simulink model "mc2_current"  (R2023b)
settings: Solver=ode45  StartTime=0.0  StopTime=0.05  MaxStep=1e-5  RelTol=1e-3
libraries: simulink x1, spsDCVoltageSourceLib x1, spsUniversalBridgeLib x1, spsVoltageMeasurementLib x1, sps_lib x1
settings Model: Creator=86189  LastModifiedBy=86189

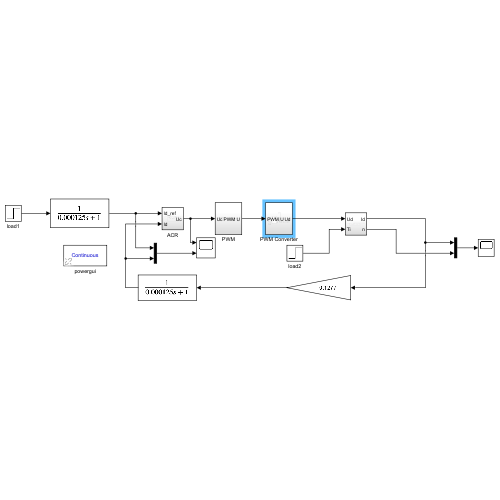
[thumbnail: Simulink's stored preview of the top-level diagram]
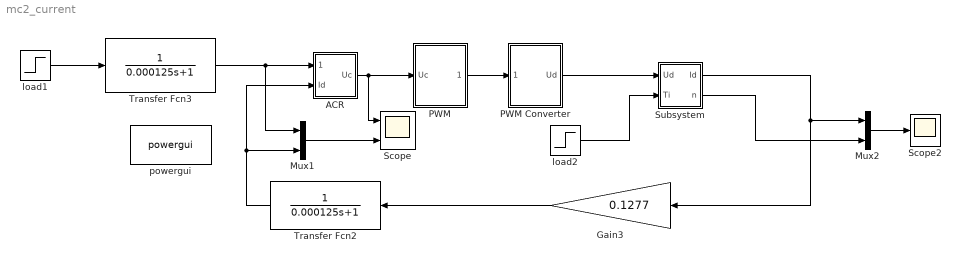
== system mc2_current ==
  ACR : Subsystem
  Gain3 : Gain  Gain=0.1277
  Mux1 : Mux  Inputs=2
  Mux2 : Mux  Inputs=2
  PWM : Subsystem
  PWM Converter : Subsystem
  Scope : Scope  NumInputPorts=2
  Scope2 : Scope
  Subsystem : Subsystem
  Transfer Fcn2 : TransferFcn  Denominator=[0.000125 1]
  Transfer Fcn3 : TransferFcn  Denominator=[0.000125 1]
  load1 : Step  Time=0  After=10  SampleTime=0
  load2 : Step  Time=0  After=10  SampleTime=0
  powergui : sps_lib/powergui  Priority=1  SimulationMode=Continuous  SampleTime=50e-6  frequency=60  Iterations=50  frequencyindice=0  Pbase=100e6  ErrMax=1e-4  UnitsV=kV  UnitsW=MW  buscounter=0  FunctionMessages=off  echomessages=off  EnableUseOfTLC=off  CurrentSourceSwitches=off  DisableSnubberDevices=off  DisableRonSwitches=off  DisableVfSwitches=off  DisplayEquations=off  AutomaticDiscreteSolvers=off  SolverType=Tustin/Backward Euler (TBE)  Interpol=off  ExternalGateDelay=off  methode=off  Ts=100  x0status=blocks  SPID=on  SwTol=0  HookPort=off  NonlinearTolerance=1e-4  nMaxIteration=100  ContinueOnMaxIteration=off  RestoreLinks=warning  ResistiveCurrentMeasurement=off  Frange=[0:2:500]  Ylog=off  Xlog=on  ShowGrid=off  save=off  variable=ZData  structure=0  ZoomFFT=off  StartTime=0.0  cycles=1  DisplayStyle=1  fundamental=60  FreqAxis=off  MaxFrequency=1000  frequencyindicesteady=1  RmsSteady=1  display=off
  wires:
  load1/1 -> Transfer Fcn3/1
  Gain3/1 -> Transfer Fcn2/1
  PWM Converter/1(Ud) -> Subsystem/1(Ud)
  Subsystem/1(Id) -> Mux2/1, Gain3/1
  load2/1 -> Subsystem/2(Ti)
  PWM/1(PWM U) -> PWM Converter/1(PWM U)
  Transfer Fcn3/1 -> Mux1/1, ACR/1(Id_ref)
  Transfer Fcn2/1 -> Mux1/2, ACR/2(Id)
  ACR/1(Uc) -> Scope/1, PWM/1(Uc)
  Mux1/1 -> Scope/2
  Subsystem/2(n) -> Mux2/2
  Mux2/1 -> Scope2/1

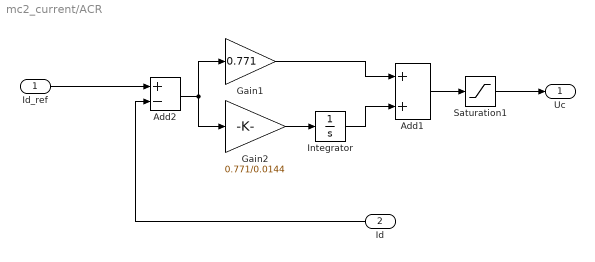
== system mc2_current/ACR ==
  Id_ref : Inport
  Id : Inport  Port=2
  Add1 : Sum
  Add2 : Sum  Inputs=+-
  Gain1 : Gain  Gain=0.771
  Gain2 : Gain  Gain=0.771/0.0144
  Integrator : Integrator  LimitOutput=on  UpperSaturationLimit=5  LowerSaturationLimit=-5
  Saturation1 : Saturate  UpperLimit=5  LowerLimit=-5
  Uc : Outport
  wires:
  Gain2/1 -> Integrator/1
  Add1/1 -> Saturation1/1
  Integrator/1 -> Add1/2
  Add2/1 -> Gain2/1, Gain1/1
  Gain1/1 -> Add1/1
  Id/1 -> Add2/2
  Id_ref/1 -> Add2/1
  Saturation1/1 -> Uc/1

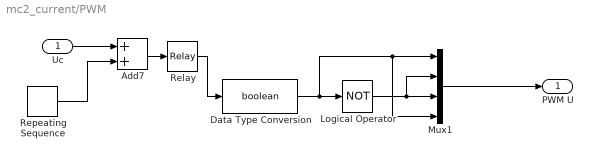
== system mc2_current/PWM ==
  Uc : Inport
  Add7 : Sum
  Data Type Conversion : DataTypeConversion  OutDataTypeStr=boolean  SaturateOnIntegerOverflow=off  RndMeth=Floor
  Logical Operator : Logic  Operator=NOT  AllPortsSameDT=off  OutDataTypeStr=boolean
  Mux1 : Mux
      settings: DisplayOption=signals
  Relay : Relay  OnSwitchValue=0  OffSwitchValue=0
  Repeating Sequence : simulink/Sources/Repeating Sequence  rep_seq_t=[0 0.125e-3]  rep_seq_y=[-5 5]
  PWM U : Outport
  wires:
  Repeating Sequence/1 -> Add7/2
  Data Type Conversion/1 -> Mux1/4, Mux1/1, Logical Operator/1
  Logical Operator/1 -> Mux1/2, Mux1/3
  Add7/1 -> Relay/1
  Mux1/1 -> PWM U/1
  Relay/1 -> Data Type Conversion/1
  Uc/1 -> Add7/1

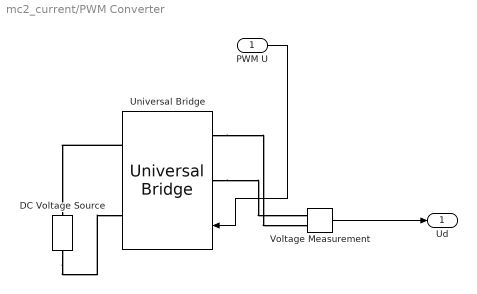
== system mc2_current/PWM Converter ==
  PWM U : Inport
  DC Voltage Source : spsDCVoltageSourceLib/DC Voltage Source  Amplitude=538  Measurements=None
  Universal Bridge : spsUniversalBridgeLib/Universal Bridge  Arms=2  SnubberResistance=1e5  SnubberCapacitance=inf  Device=MOSFET / Diodes  Ron=1e-3  Lon=0  ForwardVoltages="[  0  0  ]"  ForwardVoltage=0  GTOparameters=[ 10e-6 , 20e-6 ]  IGBTparameters=[ 1e-6 , 2e-6 ]  Measurements=None  Measurements_2=None  converterType=Rectifier
  Voltage Measurement : spsVoltageMeasurementLib/Voltage Measurement  PhasorSimulation=off  OutputType=Complex  PSBequivalent=0
  Ud : Outport
  wires:
  PWM U/1 -> Universal Bridge/1
  Voltage Measurement/1 -> Ud/1
  connections:
  Universal Bridge/LConn2 -- Voltage Measurement/LConn2
  Universal Bridge/LConn1 -- Voltage Measurement/LConn1
  DC Voltage Source/RConn1 -- Universal Bridge/RConn1
  Universal Bridge/RConn2 -- DC Voltage Source/LConn1

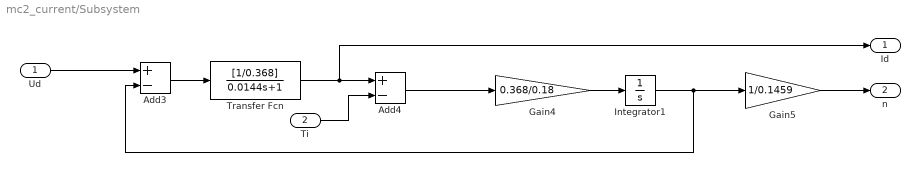
== system mc2_current/Subsystem ==
  Ud : Inport
  Ti : Inport  Port=2
  Add3 : Sum  Inputs=+-
  Add4 : Sum  Inputs=+-
  Gain4 : Gain  Gain=0.368/0.18
  Gain5 : Gain  Gain=1/0.1459
  Integrator1 : Integrator
  Transfer Fcn : TransferFcn  Numerator=[1/0.368]  Denominator=[0.0144 1]
  Id : Outport
  n : Outport  Port=2
  wires:
  Add3/1 -> Transfer Fcn/1
  Transfer Fcn/1 -> Id/1, Add4/1
  Ud/1 -> Add3/1
  Add4/1 -> Gain4/1
  Integrator1/1 -> Add3/2, Gain5/1
  Gain4/1 -> Integrator1/1
  Gain5/1 -> n/1
  Ti/1 -> Add4/2
